simulink model "f18nlclp"  (Simulink 7.2)
settings: Solver=ode45  StartTime=0.0  StopTime=10.0  RelTol=1e-3
values from neighbouring files (symbols this model uses):
  aytrim = double(subs(C(1,:)*x + D(1,:)*u,[x;u],[xtf(2:7);utf(1:3)]))    [RunF18NomSimClp.m]    (also in RunF18Sim.m = C(1,:)*xtrim(2:7) + D(1,:)*utrim(1:3))
  bdottrim = double(subs(C(end,:)*x + D(end,:)*u,[x;u],[xtf(2:7);utf(1:3)]))    [RunF18NomSimClp.m]    (also in RunF18Sim.m = C(end,:)*xtrim(2:7) + D(end,:)*utrim(1:3))
  C = Pss.C    [RunF18NomSimClp.m]    (also in RunF18Sim.m = Bank25.Pss.C)
  D = Pss.D    [RunF18NomSimClp.m]    (also in RunF18Sim.m = Bank25.Pss.D)
  K = CssR    [RunF18NomSimClp.m]    (also in RunF18Sim.m = Bank25.CssR)
  utrim = [-0.00218308158555 -0.0062308112469 -0.0468365436458 14500.0001078]    [F18Model_Coord_Phi_10.mat]    (also in F18Model_UnCoord_Phi_25.mat = [0.239553480817 0.195781713468 -0.0629449706924 14499.999992; RunF18Sim.m = Bank25.utrim)
  xtf = xtrim    [RunF18NomSimClp.m]
settings Model: Creator=chakrab  LastModifiedBy=chakrab

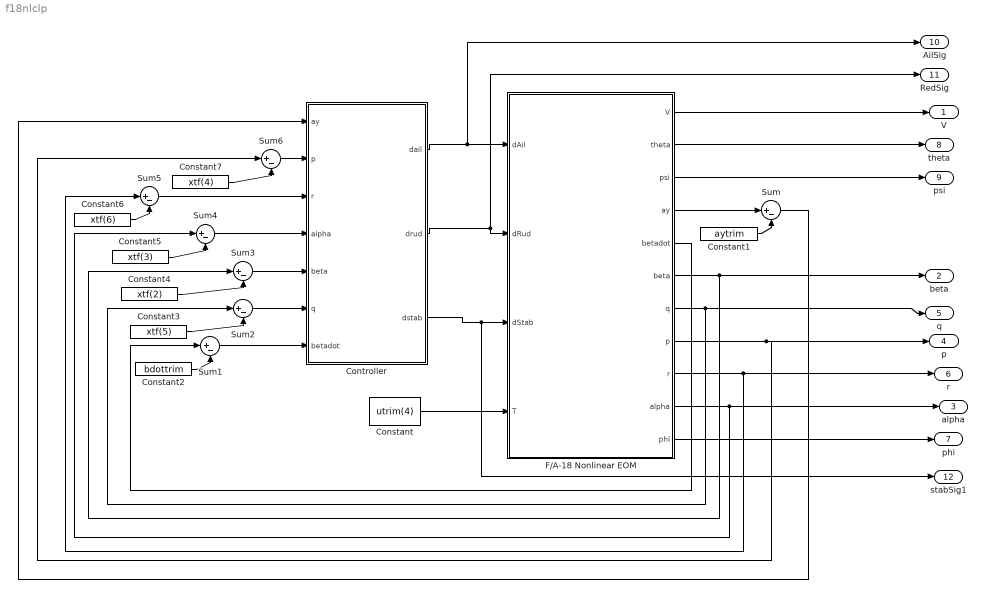
== system f18nlclp ==
  Constant : Constant  Value=utrim(4)  OutDataType=sfix(16)  OutScaling=2^0
  Constant1 : Constant  Value=aytrim  OutDataType=sfix(16)  OutScaling=2^0
  Constant2 : Constant  Value=bdottrim  OutDataType=sfix(16)  OutScaling=2^0
  Constant3 : Constant  Value=xtf(5)  OutDataType=sfix(16)  OutScaling=2^0
  Constant4 : Constant  Value=xtf(2)  OutDataType=sfix(16)  OutScaling=2^0
  Constant5 : Constant  Value=xtf(3)  OutDataType=sfix(16)  OutScaling=2^0
  Constant6 : Constant  Value=xtf(6)  OutDataType=sfix(16)  OutScaling=2^0
  Constant7 : Constant  Value=xtf(4)  OutDataType=sfix(16)  OutScaling=2^0
  Controller : Subsystem
  F/A-18 Nonlinear EOM : Subsystem
  Sum{,1..6} (7 alike) : Sum  Inputs=|+-  OutDataType=sfix(16)  OutScaling=2^0
  V : Outport  OutDataType=sfix(16)  OutScaling=2^0
  beta : Outport  Port=2  OutDataType=sfix(16)  OutScaling=2^0
  alpha : Outport  Port=3  OutDataType=sfix(16)  OutScaling=2^0
  p : Outport  Port=4  OutDataType=sfix(16)  OutScaling=2^0
  q : Outport  Port=5  OutDataType=sfix(16)  OutScaling=2^0
  r : Outport  Port=6  OutDataType=sfix(16)  OutScaling=2^0
  phi : Outport  Port=7  OutDataType=sfix(16)  OutScaling=2^0
  theta : Outport  Port=8  OutDataType=sfix(16)  OutScaling=2^0
  psi : Outport  Port=9  OutDataType=sfix(16)  OutScaling=2^0
  AilSig : Outport  Port=10  OutDataType=sfix(16)  OutScaling=2^0
  RedSig : Outport  Port=11  OutDataType=sfix(16)  OutScaling=2^0
  stabSig1 : Outport  Port=12  OutDataType=sfix(16)  OutScaling=2^0
  wires:
  Constant/1 -> F/A-18 Nonlinear EOM/4(T)
  Controller/2(drud) -> F/A-18 Nonlinear EOM/2(dRud), RedSig/1
  Controller/3(dstab) -> F/A-18 Nonlinear EOM/3(dStab), stabSig1/1
  F/A-18 Nonlinear EOM/8(p) -> p/1, Sum6/1
  F/A-18 Nonlinear EOM/9(r) -> r/1, Sum5/1
  F/A-18 Nonlinear EOM/10(alpha) -> alpha/1, Sum4/1
  F/A-18 Nonlinear EOM/6(beta) -> beta/1, Sum3/1
  F/A-18 Nonlinear EOM/7(q) -> q/1, Sum2/1
  F/A-18 Nonlinear EOM/1(V) -> V/1
  F/A-18 Nonlinear EOM/2(theta) -> theta/1
  F/A-18 Nonlinear EOM/3(psi) -> psi/1
  F/A-18 Nonlinear EOM/11(phi) -> phi/1
  Controller/1(dail) -> F/A-18 Nonlinear EOM/1(dAil), AilSig/1
  F/A-18 Nonlinear EOM/4(ay) -> Sum/1
  Sum/1 -> Controller/1(ay)
  Constant1/1 -> Sum/2
  Sum1/1 -> Controller/7(betadot)
  F/A-18 Nonlinear EOM/5(betadot) -> Sum1/1
  Constant2/1 -> Sum1/2
  Constant3/1 -> Sum2/2
  Sum2/1 -> Controller/6(q)
  Constant4/1 -> Sum3/2
  Sum3/1 -> Controller/5(beta)
  Constant5/1 -> Sum4/2
  Sum4/1 -> Controller/4(alpha)
  Constant6/1 -> Sum5/2
  Sum5/1 -> Controller/3(r)
  Sum6/1 -> Controller/2(p)
  Constant7/1 -> Sum6/2

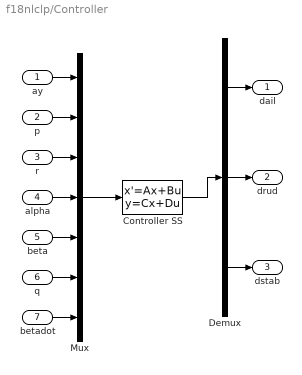
== system f18nlclp/Controller ==
  ay : Inport
  p : Inport  Port=2
  r : Inport  Port=3
  alpha : Inport  Port=4
  beta : Inport  Port=5
  q : Inport  Port=6
  betadot : Inport  Port=7
  Controller SS : StateSpace  A=K.A  B=-K.B  C=K.C  D=-K.D
  Demux : Demux  Outputs=3
  Mux : Mux  Inputs=7
  dail : Outport
  drud : Outport  Port=2
  dstab : Outport  Port=3
  wires:
  Controller SS/1 -> Demux/1
  Mux/1 -> Controller SS/1
  ay/1 -> Mux/1
  Demux/1 -> dail/1
  p/1 -> Mux/2
  r/1 -> Mux/3
  Demux/2 -> drud/1
  alpha/1 -> Mux/4
  beta/1 -> Mux/5
  Demux/3 -> dstab/1
  q/1 -> Mux/6
  betadot/1 -> Mux/7

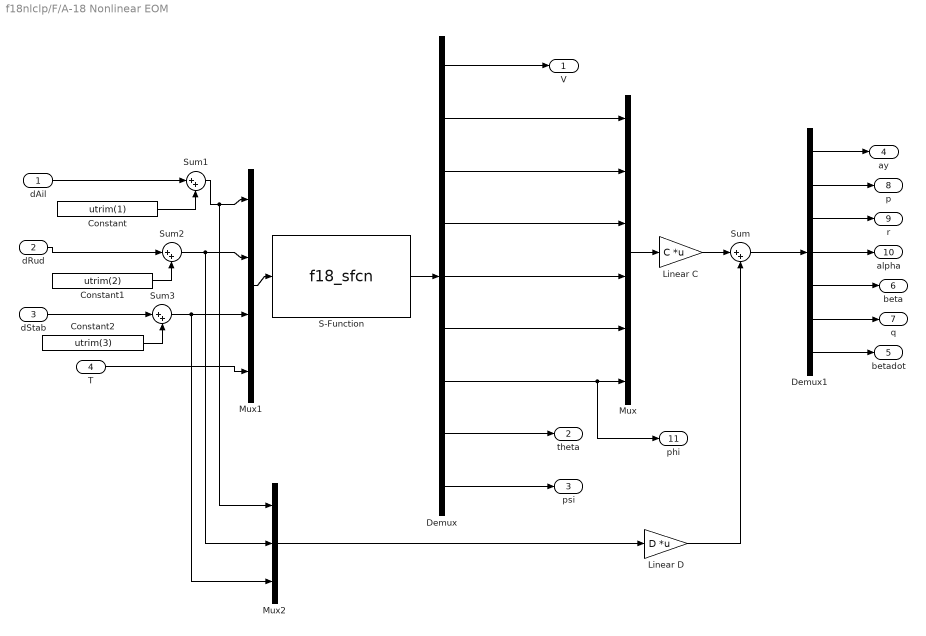
== system f18nlclp/F/A-18 Nonlinear EOM ==
  dAil : Inport
  dRud : Inport  Port=2
  dStab : Inport  Port=3
  T : Inport  Port=4
  Constant : Constant  Value=utrim(1)  OutDataType=sfix(16)  OutScaling=2^0
  Constant1 : Constant  Value=utrim(2)  OutDataType=sfix(16)  OutScaling=2^0
  Constant2 : Constant  Value=utrim(3)  OutDataType=sfix(16)  OutScaling=2^0
  Demux : Demux  Outputs=9
  Demux1 : Demux  Outputs=7
  Linear C : Gain  Gain=C  Multiplication=Matrix(K*u)  ParameterDataType=sfix(16)  ParameterScaling=2^0  OutDataType=sfix(16)  OutScaling=2^0
  Linear D : Gain  Gain=D  Multiplication=Matrix(K*u)  ParameterDataType=sfix(16)  ParameterScaling=2^0  OutDataType=sfix(16)  OutScaling=2^0
  Mux : Mux  Inputs=6
  Mux1 : Mux
  Mux2 : Mux  Inputs=3
  S-Function : S-Function  FunctionName=f18_sfcn  Parameters=dx0 , opts  EnableBusSupport=off
  Sum{,1..3} (4 alike) : Sum  Inputs=|++  OutDataType=sfix(16)  OutScaling=2^0
  V : Outport
  theta : Outport  Port=2
  psi : Outport  Port=3
  ay : Outport  Port=4  OutDataType=sfix(16)  OutScaling=2^0
  betadot : Outport  Port=5  OutDataType=sfix(16)  OutScaling=2^0
  beta : Outport  Port=6
  q : Outport  Port=7
  p : Outport  Port=8
  r : Outport  Port=9
  alpha : Outport  Port=10
  phi : Outport  Port=11
  wires:
  Mux1/1 -> S-Function/1
  S-Function/1 -> Demux/1
  Demux/1 -> V/1
  Demux/5 -> Mux/4
  Demux/2 -> Mux/1
  Demux/3 -> Mux/2
  Demux/4 -> Mux/3
  Demux/6 -> Mux/5
  T/1 -> Mux1/4
  Demux/7 -> Mux/6, phi/1
  Demux/8 -> theta/1
  Demux/9 -> psi/1
  Mux/1 -> Linear C/1
  Mux2/1 -> Linear D/1
  Linear C/1 -> Sum/1
  Linear D/1 -> Sum/2
  Sum/1 -> Demux1/1
  Demux1/1 -> ay/1
  Demux1/7 -> betadot/1
  Demux1/6 -> q/1
  Demux1/5 -> beta/1
  Demux1/2 -> p/1
  Demux1/3 -> r/1
  Demux1/4 -> alpha/1
  dAil/1 -> Sum1/1
  Sum1/1 -> Mux1/1, Mux2/1
  dRud/1 -> Sum2/1
  Sum2/1 -> Mux1/2, Mux2/2
  dStab/1 -> Sum3/1
  Sum3/1 -> Mux1/3, Mux2/3
  Constant/1 -> Sum1/2
  Constant1/1 -> Sum2/2
  Constant2/1 -> Sum3/2
